simulink model "ES002A_McuDiagc"  (R2013b)
settings: Solver=FixedStepDiscrete  SolverMode=SingleTasking  StartTime=0.0  StopTime=1  FixedStep=0.000125  RelTol=1e-3
values from neighbouring files (symbols this model uses):
  dMcuDiagcFastLoopCntrMax = DataDict.Display    [ES002A_McuDiagc_DataDict.m]
  dMcuDiagcFastLoopCntrMin = DataDict.Display    [ES002A_McuDiagc_DataDict.m]
  dMcuDiagcLoopCntr2MilliSecMotCtrlDif = DataDict.Display    [ES002A_McuDiagc_DataDict.m]
  FastLoopCntr = DataDict.IpSignal    [ES002A_McuDiagc_DataDict.m]
  FASTLOOPCNTRMAX_CNT_U08 = DataDict.Constant    [ES002A_McuDiagc_DataDict.m]
  FASTLOOPCNTRMIN_CNT_U08 = DataDict.Constant    [ES002A_McuDiagc_DataDict.m]
  FastLoopCntrPrev = DataDict.PIM    [ES002A_McuDiagc_DataDict.m]
  LOOPCNTR2MILLISECMOTCTRLCOMPPRM_CNT_U08 = DataDict.Constant    [ES002A_McuDiagc_DataDict.m]
  LOSSMOTCTRLLOOPPRM_CNT_U08 = DataDict.Constant    [ES002A_McuDiagc_DataDict.m]
  McuDiagc2MilliSecCntrCompThd = DataDict.Calibration    [ES002A_McuDiagc_DataDict.m]
  McuDiagcFlt = DataDict.NTC    [ES002A_McuDiagc_DataDict.m]
  McuDiagcFltFailStep = DataDict.Calibration    [ES002A_McuDiagc_DataDict.m]
  McuDiagcFltPassStep = DataDict.Calibration    [ES002A_McuDiagc_DataDict.m]
  MOTCTRLDIAGCINITDLY_CNT_U08 = DataDict.Constant    [ES002A_McuDiagc_DataDict.m]
undefined symbols (not defined in the file or in its folder): NtcSts1, sigbuilder_block
libraries: simulink x10, NxtrMax x1, NxtrMin x1
(part 2 of 2)

== system ES002A_McuDiagc/McuDiagc/McuDiagcPer2/Diagnose Fault Loop Counter/Calculate LoopCntrDelta/Counter Rolled Over ==
  FastLoopCntr : Inport
  LoopCntrPrev : Inport  Port=2
  Action Port : ActionPort  ActionType=else
  Bias : Bias  Bias=1.0
  CopyRight2 : Subsystem  Description=|  mask(Copyright Information){none=on}
      | Copyright info block.                                               
      |                                                                     
      | Place copyright information at the top of every subsystem in design.
      mask prompts: none "No parameters"
      mask help: Place copyright information at the top of every subsystem in design.
      mask Display:
      | NxtrConf = 'Nexteer Confidential';
      | 
      | sys = bdroot; %handle for the current model ("system")
      | first = get_param(sys,'Created');
      | first = first(end-3:end);  %year is last four digits
      | 
      | last = get_param(sys,'LastModifiedDate');
      | if isempty(last)
      |     last = datestr(now,'yyyy');
      | else
      |     last = last(end-3:end);
      | end
      | 
      | if strcmp(first,last)
      |     fprintf('%s -- Copyright %s Nexteer',NxtrConf,first)
      | else
      |     fprintf('%s -- %s%s- %s Nexteer',NxtrConf,char(169),first,last)
      | end
  Data Type Conversion2 : DataTypeConversion  OutMin=0  OutMax=65535  OutDataTypeStr=uint16
  FLTINJ_CURRMEAS_MOTCURRCORRDA2 : Constant  Value=FastLoopCntr.EngMax  OutDataTypeStr=uint32
  Subtract : Sum  Inputs=+-
  Subtract1 : Sum
  LoopCntrDelta : Outport
  wires:
  Subtract/1 -> Subtract1/1
  FLTINJ_CURRMEAS_MOTCURRCORRDA2/1 -> Data Type Conversion2/1
  LoopCntrPrev/1 -> Subtract/2
  FastLoopCntr/1 -> Subtract1/2
  Subtract1/1 -> Bias/1
  Data Type Conversion2/1 -> Subtract/1
  Bias/1 -> LoopCntrDelta/1

== system ES002A_McuDiagc/McuDiagc/McuDiagcPer2/Diagnose Fault Loop Counter/Calculate LoopCntrDelta/No Rollover Condition ==
  FastLoopCntr : Inport
  LoopCntrPrev : Inport  Port=2
  Action Port : ActionPort  ActionType=then
  CopyRight2 : Subsystem  Description=|  mask(Copyright Information){none=on}
      | Copyright info block.                                               
      |                                                                     
      | Place copyright information at the top of every subsystem in design.
      mask prompts: none "No parameters"
      mask help: Place copyright information at the top of every subsystem in design.
      mask Display:
      | NxtrConf = 'Nexteer Confidential';
      | 
      | sys = bdroot; %handle for the current model ("system")
      | first = get_param(sys,'Created');
      | first = first(end-3:end);  %year is last four digits
      | 
      | last = get_param(sys,'LastModifiedDate');
      | if isempty(last)
      |     last = datestr(now,'yyyy');
      | else
      |     last = last(end-3:end);
      | end
      | 
      | if strcmp(first,last)
      |     fprintf('%s -- Copyright %s Nexteer',NxtrConf,first)
      | else
      |     fprintf('%s -- %s%s- %s Nexteer',NxtrConf,char(169),first,last)
      | end
  Subtract : Sum  Inputs=+-
  LoopCntrDelta : Outport
  wires:
  FastLoopCntr/1 -> Subtract/1
  LoopCntrPrev/1 -> Subtract/2
  Subtract/1 -> LoopCntrDelta/1

== system ES002A_McuDiagc/McuDiagc/McuDiagcPer2/Diagnose Fault Loop Counter/Capture Min Max Delta/CopyRight2 ==

== system ES002A_McuDiagc/McuDiagc/McuDiagcPer2/Diagnose Fault Loop Counter/Determine difference b//w 2ms loop cntr and MotCtrlISR version of 2ms loop cntr/Capture Max Dif ==
  LoopCntr2MilliSecMotCtrlDif : Inport
  CopyRight2 : Subsystem  Description=|  mask(Copyright Information){none=on}
      | Copyright info block.                                               
      |                                                                     
      | Place copyright information at the top of every subsystem in design.
      mask prompts: none "No parameters"
      mask help: Place copyright information at the top of every subsystem in design.
      mask Display:
      | NxtrConf = 'Nexteer Confidential';
      | 
      | sys = bdroot; %handle for the current model ("system")
      | first = get_param(sys,'Created');
      | first = first(end-3:end);  %year is last four digits
      | 
      | last = get_param(sys,'LastModifiedDate');
      | if isempty(last)
      |     last = datestr(now,'yyyy');
      | else
      |     last = last(end-3:end);
      | end
      | 
      | if strcmp(first,last)
      |     fprintf('%s -- Copyright %s Nexteer',NxtrConf,first)
      | else
      |     fprintf('%s -- %s%s- %s Nexteer',NxtrConf,char(169),first,last)
      | end
  Data Store Read : DataStoreRead  DataStoreName=dMcuDiagcLoopCntr2MilliSecMotCtrlDif
  Data Store Write : DataStoreWrite  DataStoreName=dMcuDiagcLoopCntr2MilliSecMotCtrlDif
  Display1 : Display
  MinMax : MinMax  Function=max  Inputs=2
  wires:
  LoopCntr2MilliSecMotCtrlDif/1 -> MinMax/1
  MinMax/1 -> Display1/1, Data Store Write/1
  Data Store Read/1 -> MinMax/2

== system ES002A_McuDiagc/McuDiagc/McuDiagcPer2/Diagnose Fault Loop Counter/Determine difference b//w 2ms loop cntr and MotCtrlISR version of 2ms loop cntr/Compare 2ms Loop Cntr to MotCtrl ISR ==
  LoopCntr2MilliSecDelta : Inport
  Action Port : ActionPort  ActionType=else
  Constant : Constant  Description=|  Value=65535  OutDataTypeStr=uint16
      | Data Type max of 
      | LoopCnt2MilliSecIntRun 
      | and SlowLoopCntr
      settings: AttributesFormatString=%<Description>
  CopyRight2 : Subsystem  Description=|  mask(Copyright Information){none=on}
      | Copyright info block.                                               
      |                                                                     
      | Place copyright information at the top of every subsystem in design.
      mask prompts: none "No parameters"
      mask help: Place copyright information at the top of every subsystem in design.
      mask Display:
      | NxtrConf = 'Nexteer Confidential';
      | 
      | sys = bdroot; %handle for the current model ("system")
      | first = get_param(sys,'Created');
      | first = first(end-3:end);  %year is last four digits
      | 
      | last = get_param(sys,'LastModifiedDate');
      | if isempty(last)
      |     last = datestr(now,'yyyy');
      | else
      |     last = last(end-3:end);
      | end
      | 
      | if strcmp(first,last)
      |     fprintf('%s -- Copyright %s Nexteer',NxtrConf,first)
      | else
      |     fprintf('%s -- %s%s- %s Nexteer',NxtrConf,char(169),first,last)
      | end
  Subtract : Sum  Inputs=+-
  LoopCntr2MilliSecMotCtrlDif : Outport
  wires:
  LoopCntr2MilliSecDelta/1 -> Subtract/2
  Constant/1 -> Subtract/1
  Subtract/1 -> LoopCntr2MilliSecMotCtrlDif/1

== system ES002A_McuDiagc/McuDiagc/McuDiagcPer2/Diagnose Fault Loop Counter/Determine difference b//w 2ms loop cntr and MotCtrlISR version of 2ms loop cntr/Compare 2ms Loop Cntr to MotCtrl ISR1 ==
  LoopCntr2MilliSecDelta : Inport
  Action Port : ActionPort  ActionType=then
  CopyRight2 : Subsystem  Description=|  mask(Copyright Information){none=on}
      | Copyright info block.                                               
      |                                                                     
      | Place copyright information at the top of every subsystem in design.
      mask prompts: none "No parameters"
      mask help: Place copyright information at the top of every subsystem in design.
      mask Display:
      | NxtrConf = 'Nexteer Confidential';
      | 
      | sys = bdroot; %handle for the current model ("system")
      | first = get_param(sys,'Created');
      | first = first(end-3:end);  %year is last four digits
      | 
      | last = get_param(sys,'LastModifiedDate');
      | if isempty(last)
      |     last = datestr(now,'yyyy');
      | else
      |     last = last(end-3:end);
      | end
      | 
      | if strcmp(first,last)
      |     fprintf('%s -- Copyright %s Nexteer',NxtrConf,first)
      | else
      |     fprintf('%s -- %s%s- %s Nexteer',NxtrConf,char(169),first,last)
      | end
  LoopCntr2MilliSecMotCtrlDif : Outport
  wires:
  LoopCntr2MilliSecDelta/1 -> LoopCntr2MilliSecMotCtrlDif/1

== system ES002A_McuDiagc/McuDiagc/McuDiagcPer2/Diagnose Fault Loop Counter/Determine difference b//w 2ms loop cntr and MotCtrlISR version of 2ms loop cntr/CopyRight2 ==

== system ES002A_McuDiagc/McuDiagc/McuDiagcPer2/Diagnose Fault Loop Counter/Fault Determination/CopyRight2 ==

== system ES002A_McuDiagc/McuDiagc/McuDiagcPer2/Diagnose Fault Loop Counter/Fault Determination/NTC Fault Processing ==
  NtcStInfo : Inport  OutDataTypeStr=uint8
  Action Port : ActionPort  ActionType=then
  Calibration : Constant  Value=McuDiagcFltFailStep
  Constant3 : Constant  Value=McuDiagcFlt
  CopyRight2 : Subsystem  Description=|  mask(Copyright Information){none=on}
      | Copyright info block.                                               
      |                                                                     
      | Place copyright information at the top of every subsystem in design.
      mask prompts: none "No parameters"
      mask help: Place copyright information at the top of every subsystem in design.
      mask Display:
      | NxtrConf = 'Nexteer Confidential';
      | 
      | sys = bdroot; %handle for the current model ("system")
      | first = get_param(sys,'Created');
      | first = first(end-3:end);  %year is last four digits
      | 
      | last = get_param(sys,'LastModifiedDate');
      | if isempty(last)
      |     last = datestr(now,'yyyy');
      | else
      |     last = last(end-3:end);
      | end
      | 
      | if strcmp(first,last)
      |     fprintf('%s -- Copyright %s Nexteer',NxtrConf,first)
      | else
      |     fprintf('%s -- %s%s- %s Nexteer',NxtrConf,char(169),first,last)
      | end
  NtcNr1 : simulink/Sources/Enumerated Constant  OutDataTypeStr=Enum: NtcSts1  Value=NtcSts1.NTCSTS_PREFAILD  SampleTime=inf
  SetNtcSts : Subsystem
  wires:
  Constant3/1 -> SetNtcSts/1(NtcNr)
  NtcNr1/1 -> SetNtcSts/3(NtcSts)
  Calibration/1 -> SetNtcSts/4(DebStep)
  NtcStInfo/1 -> SetNtcSts/2(NtcStInfo)

== system ES002A_McuDiagc/McuDiagc/McuDiagcPer2/Diagnose Fault Loop Counter/Fault Determination/Pass Diagc ==
  Action Port : ActionPort  ActionType=else
  Calibration : Constant  Value=McuDiagcFltPassStep  OutDataTypeStr=uint16
  Constant3 : Constant  Value=McuDiagcFlt
  CopyRight2 : Subsystem  Description=|  mask(Copyright Information){none=on}
      | Copyright info block.                                               
      |                                                                     
      | Place copyright information at the top of every subsystem in design.
      mask prompts: none "No parameters"
      mask help: Place copyright information at the top of every subsystem in design.
      mask Display:
      | NxtrConf = 'Nexteer Confidential';
      | 
      | sys = bdroot; %handle for the current model ("system")
      | first = get_param(sys,'Created');
      | first = first(end-3:end);  %year is last four digits
      | 
      | last = get_param(sys,'LastModifiedDate');
      | if isempty(last)
      |     last = datestr(now,'yyyy');
      | else
      |     last = last(end-3:end);
      | end
      | 
      | if strcmp(first,last)
      |     fprintf('%s -- Copyright %s Nexteer',NxtrConf,first)
      | else
      |     fprintf('%s -- %s%s- %s Nexteer',NxtrConf,char(169),first,last)
      | end
  Dummy Param Byte : Constant  Value=0  OutDataTypeStr=uint8
  NtcNr1 : simulink/Sources/Enumerated Constant  OutDataTypeStr=Enum: NtcSts1  Value=NtcSts1.NTCSTS_PREPASSD  SampleTime=inf
  SetNtcSts : Subsystem
  wires:
  Constant3/1 -> SetNtcSts/1(NtcNr)
  Dummy Param Byte/1 -> SetNtcSts/2(NtcStInfo)
  NtcNr1/1 -> SetNtcSts/3(NtcSts)
  Calibration/1 -> SetNtcSts/4(DebStep)

== system ES002A_McuDiagc/McuDiagc/McuDiagcPer2/Diagnose Fault Loop Counter/Motor Control Loop counter diagnosis/CopyRight2 ==

== system ES002A_McuDiagc/McuDiagc/McuDiagcPer2/Diagnose Fault Loop Counter/Calculate LoopCntrDelta/Counter Rolled Over/CopyRight2 ==

== system ES002A_McuDiagc/McuDiagc/McuDiagcPer2/Diagnose Fault Loop Counter/Calculate LoopCntrDelta/No Rollover Condition/CopyRight2 ==

== system ES002A_McuDiagc/McuDiagc/McuDiagcPer2/Diagnose Fault Loop Counter/Determine difference b//w 2ms loop cntr and MotCtrlISR version of 2ms loop cntr/Capture Max Dif/CopyRight2 ==

== system ES002A_McuDiagc/McuDiagc/McuDiagcPer2/Diagnose Fault Loop Counter/Determine difference b//w 2ms loop cntr and MotCtrlISR version of 2ms loop cntr/Compare 2ms Loop Cntr to MotCtrl ISR/CopyRight2 ==

== system ES002A_McuDiagc/McuDiagc/McuDiagcPer2/Diagnose Fault Loop Counter/Determine difference b//w 2ms loop cntr and MotCtrlISR version of 2ms loop cntr/Compare 2ms Loop Cntr to MotCtrl ISR1/CopyRight2 ==

== system ES002A_McuDiagc/McuDiagc/McuDiagcPer2/Diagnose Fault Loop Counter/Fault Determination/NTC Fault Processing/CopyRight2 ==

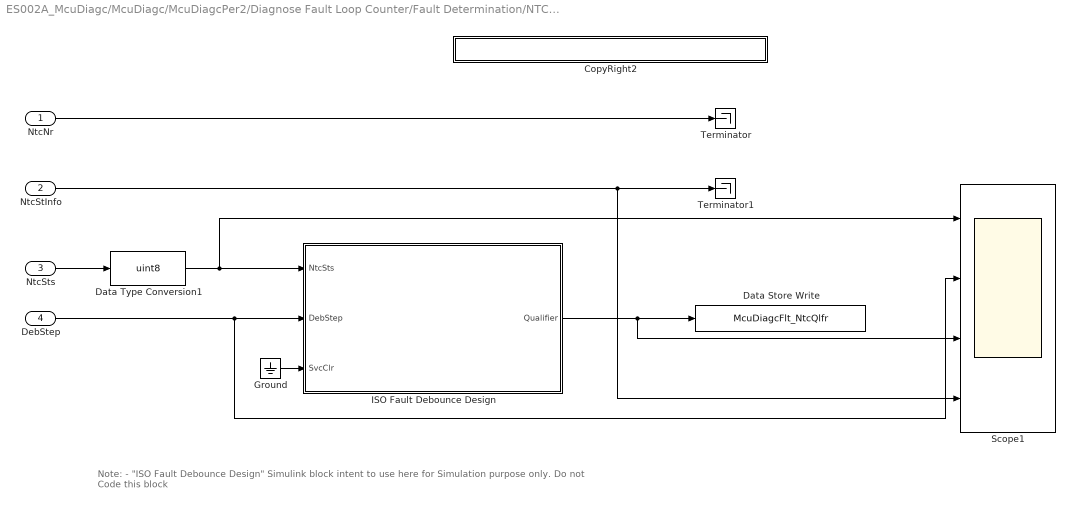
== system ES002A_McuDiagc/McuDiagc/McuDiagcPer2/Diagnose Fault Loop Counter/Fault Determination/NTC Fault Processing/SetNtcSts ==
  note: Note:
      |
      | - "ISO Fault Debounce Design" Simulink block intent to use here for Simulation purpose only. Do not Code this block
  NtcNr : Inport
  NtcStInfo : Inport  Port=2
  NtcSts : Inport  Port=3  OutDataTypeStr=Enum: NtcSts1
  DebStep : Inport  Port=4
  CopyRight2 : Subsystem  Description=|  mask(Copyright Information){none=on}
      | Copyright info block.                                               
      |                                                                     
      | Place copyright information at the top of every subsystem in design.
      mask prompts: none "No parameters"
      mask help: Place copyright information at the top of every subsystem in design.
      mask Display:
      | NxtrConf = 'Nexteer Confidential';
      | 
      | sys = bdroot; %handle for the current model ("system")
      | first = get_param(sys,'Created');
      | first = first(end-3:end);  %year is last four digits
      | 
      | last = get_param(sys,'LastModifiedDate');
      | if isempty(last)
      |     last = datestr(now,'yyyy');
      | else
      |     last = last(end-3:end);
      | end
      | 
      | if strcmp(first,last)
      |     fprintf('%s -- Copyright %s Nexteer',NxtrConf,first)
      | else
      |     fprintf('%s -- %s%s- %s Nexteer',NxtrConf,char(169),first,last)
      | end
  Data Store Write : DataStoreWrite  DataStoreName=McuDiagcFlt_NtcQlfr
  Data Type Conversion1 : DataTypeConversion  OutMin=0  OutMax=255  OutDataTypeStr=uint8
  Ground : Ground
  ISO Fault Debounce Design : Stateflow chart  TreatAsAtomicUnit=on
      settings: AttributesFormatString=|
      | Simulation Purpose Only.
      | Do Not Code this block
      | Diagnostic Manager Owns this requirement
  Scope1 : Scope  NumInputPorts=4
      settings: YMin=-5~-5~-5~-5  YMax=5~5~5~5  SaveName=ScopeData5
  Terminator : Terminator
  Terminator1 : Terminator
  wires:
  Data Type Conversion1/1 -> Scope1/1, ISO Fault Debounce Design/1(NtcSts)
  Ground/1 -> ISO Fault Debounce Design/3(SvcClr)
  ISO Fault Debounce Design/1(Qualifier) -> Data Store Write/1, Scope1/3
  DebStep/1 -> Scope1/2, ISO Fault Debounce Design/2(DebStep)
  NtcSts/1 -> Data Type Conversion1/1
  NtcNr/1 -> Terminator/1
  NtcStInfo/1 -> Terminator1/1, Scope1/4

== system ES002A_McuDiagc/McuDiagc/McuDiagcPer2/Diagnose Fault Loop Counter/Fault Determination/Pass Diagc/CopyRight2 ==

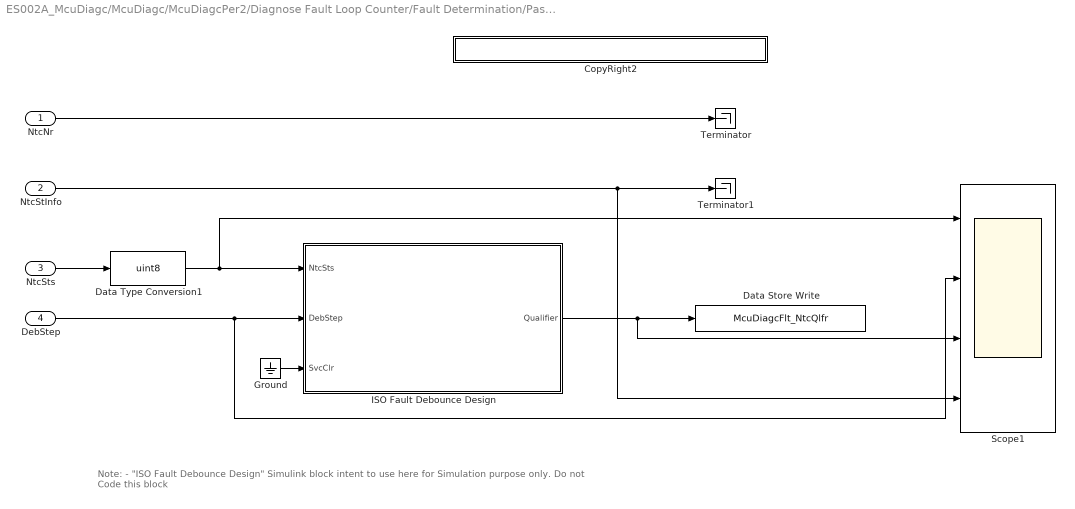
== system ES002A_McuDiagc/McuDiagc/McuDiagcPer2/Diagnose Fault Loop Counter/Fault Determination/Pass Diagc/SetNtcSts ==
  note: Note:
      |
      | - "ISO Fault Debounce Design" Simulink block intent to use here for Simulation purpose only. Do not Code this block
  NtcNr : Inport
  NtcStInfo : Inport  Port=2
  NtcSts : Inport  Port=3  OutDataTypeStr=Enum: NtcSts1
  DebStep : Inport  Port=4
  CopyRight2 : Subsystem  Description=|  mask(Copyright Information){none=on}
      | Copyright info block.                                               
      |                                                                     
      | Place copyright information at the top of every subsystem in design.
      mask prompts: none "No parameters"
      mask help: Place copyright information at the top of every subsystem in design.
      mask Display:
      | NxtrConf = 'Nexteer Confidential';
      | 
      | sys = bdroot; %handle for the current model ("system")
      | first = get_param(sys,'Created');
      | first = first(end-3:end);  %year is last four digits
      | 
      | last = get_param(sys,'LastModifiedDate');
      | if isempty(last)
      |     last = datestr(now,'yyyy');
      | else
      |     last = last(end-3:end);
      | end
      | 
      | if strcmp(first,last)
      |     fprintf('%s -- Copyright %s Nexteer',NxtrConf,first)
      | else
      |     fprintf('%s -- %s%s- %s Nexteer',NxtrConf,char(169),first,last)
      | end
  Data Store Write : DataStoreWrite  DataStoreName=McuDiagcFlt_NtcQlfr
  Data Type Conversion1 : DataTypeConversion  OutMin=0  OutMax=255  OutDataTypeStr=uint8
  Ground : Ground
  ISO Fault Debounce Design : Stateflow chart  TreatAsAtomicUnit=on
      settings: AttributesFormatString=|
      | Simulation Purpose Only.
      | Do Not Code this block
      | Diagnostic Manager Owns this requirement
  Scope1 : Scope  NumInputPorts=4
      settings: YMin=-5~-5~-5~-5  YMax=5~5~5~5  SaveName=ScopeData5
  Terminator : Terminator
  Terminator1 : Terminator
  wires:
  Data Type Conversion1/1 -> Scope1/1, ISO Fault Debounce Design/1(NtcSts)
  Ground/1 -> ISO Fault Debounce Design/3(SvcClr)
  ISO Fault Debounce Design/1(Qualifier) -> Data Store Write/1, Scope1/3
  DebStep/1 -> Scope1/2, ISO Fault Debounce Design/2(DebStep)
  NtcSts/1 -> Data Type Conversion1/1
  NtcNr/1 -> Terminator/1
  NtcStInfo/1 -> Terminator1/1, Scope1/4

== system ES002A_McuDiagc/McuDiagc/McuDiagcPer2/Diagnose Fault Loop Counter/Fault Determination/NTC Fault Processing/SetNtcSts/CopyRight2 ==

== system ES002A_McuDiagc/McuDiagc/McuDiagcPer2/Diagnose Fault Loop Counter/Fault Determination/Pass Diagc/SetNtcSts/CopyRight2 ==

== stateflow chart ES002A_McuDiagc/McuDiagc/McuDiagcPer2/Diagnose Fault Loop Counter/Fault Determination/Pass Diagc/SetNtcSts/ISO Fault Debounce Design ==
  note: NTCSTS_PASSD           (0)
      | NTCSTS_FAILD             (1)
      | NTCSTS_PREPASSD   (2)
      | NTCSTS_PREFAILD     (3)
      |
      | SIGQLFR_NORES        (0)
      | SIGQLFR_PASSD         (1)
      | SIGQLFR_FAILD           (2)
  note: Pass Loop
  note: Fail Loop
  note: 
  (default) -> (junction 89)
  (junction 89) -> (junction 95) [order 1] : [NtcSts ==3]
  (junction 89) -> (junction 93) [order 2] : [NtcSts ==2]
  (junction 89) -> (junction 141) [order 3] : [NtcSts ==1]
      | { ErrAcc = 32767;
      | Qualifier =2;
      |  }
  (junction 89) -> (junction 141) [order 4] : [NtcSts ==0]
      | { ErrAcc = -32768;
      | Qualifier=1;
      | }
  (junction 95) -> (junction 103) [order 2]
  (junction 95) -> (junction 111) [order 1] : [ErrAcc <=0]
      | {ErrAcc = DebStep;}
  (junction 93) -> (junction 123) [order 2] : {
      | ErrAcc = ErrAcc - DebStep;
      | }
  (junction 93) -> (junction 123) [order 1] : [(ErrAcc - DebStep) <= -32768]
      | { ErrAcc = -32768;
      | Qualifier=1;
      | }
  (junction 103) -> (junction 111) [order 1] : [(ErrAcc + DebStep) <32767]
      | {ErrAcc = ErrAcc + DebStep;}
  (junction 103) -> (junction 111) [order 2] : {ErrAcc = 32767;
      | Qualifier =2;}
  (junction 123) -> (junction 141)
  (junction 111) -> (junction 141)
  (junction 141) -> (junction 159) [order 2] : {ErrAcc = 0;
      | Qualifier =0;
      | }
  (junction 141) -> (junction 159) [order 1] : [SvcClr ==0]
  data: NtcSts input uint8; Qualifier output uint8; DebStep input uint16; ErrAcc local int16; SvcClr input

== stateflow chart ES002A_McuDiagc/McuDiagc/McuDiagcPer2/Diagnose Fault Loop Counter/Fault Determination/NTC Fault Processing/SetNtcSts/ISO Fault Debounce Design ==
  note: NTCSTS_PASSD           (0)
      | NTCSTS_FAILD             (1)
      | NTCSTS_PREPASSD   (2)
      | NTCSTS_PREFAILD     (3)
      |
      | SIGQLFR_NORES        (0)
      | SIGQLFR_PASSD         (1)
      | SIGQLFR_FAILD           (2)
  note: Pass Loop
  note: Fail Loop
  note: 
  (default) -> (junction 89)
  (junction 89) -> (junction 95) [order 1] : [NtcSts ==3]
  (junction 89) -> (junction 93) [order 2] : [NtcSts ==2]
  (junction 89) -> (junction 141) [order 3] : [NtcSts ==1]
      | { ErrAcc = 32767;
      | Qualifier =2;
      |  }
  (junction 89) -> (junction 141) [order 4] : [NtcSts ==0]
      | { ErrAcc = -32768;
      | Qualifier=1;
      | }
  (junction 95) -> (junction 103) [order 2]
  (junction 95) -> (junction 111) [order 1] : [ErrAcc <=0]
      | {ErrAcc = DebStep;}
  (junction 93) -> (junction 123) [order 2] : {
      | ErrAcc = ErrAcc - DebStep;
      | }
  (junction 93) -> (junction 123) [order 1] : [(ErrAcc - DebStep) <= -32768]
      | { ErrAcc = -32768;
      | Qualifier=1;
      | }
  (junction 103) -> (junction 111) [order 1] : [(ErrAcc + DebStep) <32767]
      | {ErrAcc = ErrAcc + DebStep;}
  (junction 103) -> (junction 111) [order 2] : {ErrAcc = 32767;
      | Qualifier =2;}
  (junction 123) -> (junction 141)
  (junction 111) -> (junction 141)
  (junction 141) -> (junction 159) [order 2] : {ErrAcc = 0;
      | Qualifier =0;
      | }
  (junction 141) -> (junction 159) [order 1] : [SvcClr ==0]
  data: NtcSts input uint8; Qualifier output uint8; DebStep input uint16; ErrAcc local int16; SvcClr input
